simulink library "NREL_Diesel_Genset_lib"  (Simulink 8.1)
settings: Solver=ode45  StartTime=0.0  StopTime=10.0  RelTol=1e-3
values from neighbouring files (symbols this model uses):
  T3dend = [ 1.0000   -0.9913 ]    [initGTS.m]
  T3numd = [ 0    0.0087 ]    [initGTS.m]
  T4numd = [ 27.7778  -27.7237 ]    [initGTS.m]
undefined symbols (not defined in the file or in its folder): DiscIntNeverNeededParam, Efd0, Efd1, Efd2, GP, Ka, Ke, Kf, SeEfd1, SeEfd2, Ta, Te, Tf, Ts, VR0, VRmax, VRmin
libraries: simulink x17, powerlib x9, powerlib_extras x2, powerlib_models x1
(part 2 of 2)

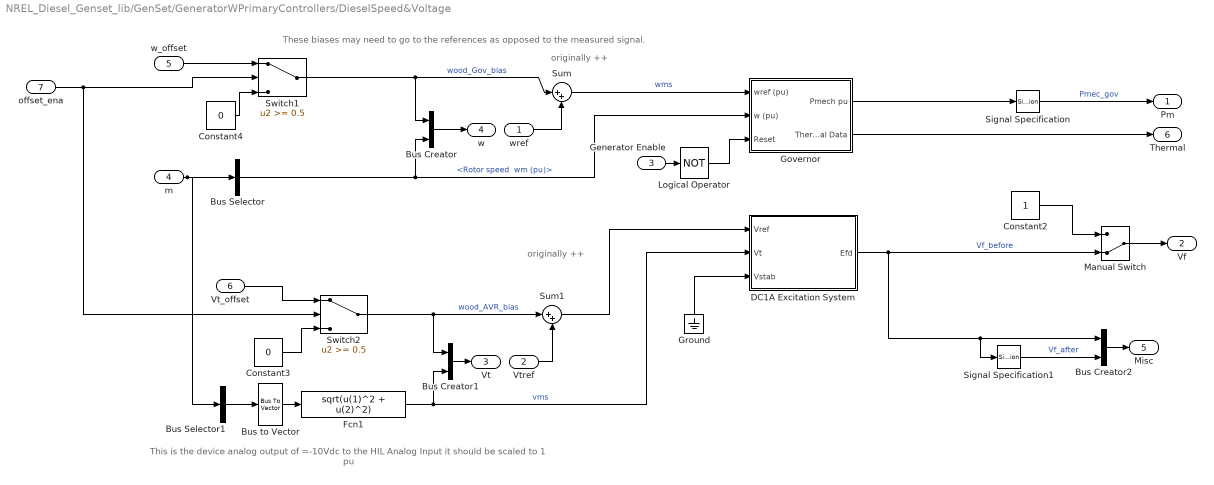
== system NREL_Diesel_Genset_lib/GenSet/GeneratorWPrimaryControllers/DieselSpeed&Voltage ==
  note: originally ++
  note: originally ++
  note: These biases may need to
      | go to the references as opposed
      | to the measured signal.
  note: This is the device analog output of =-10Vdc to
      | the HIL Analog Input it should be scaled to 1 pu
  wref : Inport  SampleTime=Ts
  Vtref : Inport  Port=2  SampleTime=Ts
  Generator Enable : Inport  Port=3  SampleTime=Ts
  m : Inport  Port=4  SampleTime=Ts
  w_offset : Inport  Port=5
  Vt_offset : Inport  Port=6
  offset_ena : Inport  Port=7
  Bus Creator : BusCreator  Inputs=2
  Bus Creator1 : BusCreator  Inputs=2
  Bus Creator2 : BusCreator  Inputs=2
  Bus Selector : BusSelector  OutputSignals="Mechanical.Rotor speed  wm (pu)"
  Bus Selector1 : BusSelector  OutputSignals="dq0 components.Stator voltage  vd (pu),dq0 components.Stator voltage  vq (pu)"  OutputAsBus=on
  Bus to Vector : BusToVector
  Constant2 : Constant
  Constant3 : Constant  Value=0
  Constant4 : Constant  Value=0
  DC1A Excitation System : Subsystem  mask(DC1A Excitation System){Tr=GP.Ex.Tr, KaTa=GP.Ex.Regulator, VRminmax=[0 8], KfTf=GP.Ex.Damping, TbTc=[0 0], KeTe=GP.Ex.Exciter, Efd12=[6.83 6.08], SeEfd12=[ 0.132 0.062], v0=[0 0], TsBlock=Ts}
      mask prompts: Tr "Low-pass filter time constant Tr(s):"; KaTa "Voltage regulator gain and time constant [Ka Ta(s)]:"; VRminmax "Voltage regulator output limits [VRmin(pu) VRmax(pu)]:"; KfTf "Damping filter gain and time constant [Kf Tf(s)]:"; TbTc "Transient gain reduction lead and lag time constants [Tb(s) Tc(s)]:"; KeTe "Exciter gain and time constant [Ke Te(s)]:"; Efd12 "Field voltage values [Efd1(pu) Efd2(pu)]:"; SeEfd12 "Exciter saturation function values [SeEfd1(pu) SeEfd2(pu)]:"; v0 "Initial values of terminal voltage and field voltage [Vt0(pu) Efd0(pu)]:"; TsBlock "Sample time:"
      mask help: Implements a synchronous machine voltage regulator and exciter based on the IEEE type DC1A excitation system model. The output is the field voltage to apply to the Vf input of a Synchronous Machine block. Inputs and output are in p.u.
      mask init:
      | block = gcb;
      | [Ts,BlockChoice,MaskType,Ka,Ta,Ke,Te,Kf,Tf,Tb,Tc,Efd1,Efd2,SeEfd1,SeEfd2,VRmin,VRmax,Vt0,Efd0,VR0] = powericon('ExcitationSystemInit',block,TsBlock,KaTa,KeTe,KfTf,TbTc,Efd12,SeEfd12,VRminmax,v0);
      | %powericon('SetInternalModels','set',block,BlockChoice);
      mask Help: helpview(psbhelp);
      mask Display: color('blue');disp('DC1A')
  Fcn1 : Fcn  Expr=sqrt(u(1)^2 + u(2)^2)
  Governor : Subsystem  BlockChoice=DieselGovernor
      settings: AttributesFormatString=%<BlockChoice>  TemplateBlock=NREL_Diesel_Genset_lib/GovernorConfig  MemberBlocks=DieselGovernor,GEJenbacherJ620
  Ground : Ground
  Logical Operator : Logic  Operator=NOT  AllPortsSameDT=off  OutDataTypeStr=boolean
  Manual Switch : ManualSwitch  CurrentSetting=0
  Signal Specification : SignalSpecification  Dimensions=1
  Signal Specification1 : SignalSpecification  Dimensions=1
  Sum : Sum  Inputs=|++
  Sum1 : Sum  Inputs=|++
  Switch1 : Switch  Threshold=0.5
  Switch2 : Switch  Threshold=0.5
  Pm : Outport
  Vf : Outport  Port=2
  Vt : Outport  Port=3
  w : Outport  Port=4
  Misc : Outport  Port=5
  Thermal : Outport  Port=6
  wires:
  Governor/2(Thermal Data) -> Thermal/1
  Governor/1(Pmech pu) -> Signal Specification/1
  Logical Operator/1 -> Governor/3(Reset)
  Signal Specification1/1 -> Bus Creator2/2  "Vf_after"
  Signal Specification/1 -> Pm/1  "Pmec_gov"
  Sum/1 -> Governor/1(wref (pu))  "wms"
  wref/1 -> Sum/2
  Sum1/1 -> DC1A Excitation System/1(Vref)
  Vtref/1 -> Sum1/2
  Switch2/1 -> Bus Creator1/1, Sum1/1  "wood_AVR_bias"
  Switch1/1 -> Bus Creator/1, Sum/1  "wood_Gov_bias"
  Bus Creator2/1 -> Misc/1
  DC1A Excitation System/1(Efd) -> Manual Switch/2, Bus Creator2/1, Signal Specification1/1  "Vf_before"
  Bus Creator1/1 -> Vt/1
  Bus Creator/1 -> w/1
  Ground/1 -> DC1A Excitation System/3(Vstab)
  Fcn1/1 -> Bus Creator1/2, DC1A Excitation System/2(Vt)  "vms"
  Bus Selector/1 -> Governor/2(w (pu)), Bus Creator/2  "<Rotor speed  wm (pu)>"
  m/1 -> Bus Selector/1, Bus Selector1/1
  Bus Selector1/1 -> Bus to Vector/1
  Bus to Vector/1 -> Fcn1/1
  Generator Enable/1 -> Logical Operator/1
  Constant2/1 -> Manual Switch/1
  Manual Switch/1 -> Vf/1
  Vt_offset/1 -> Switch2/1
  offset_ena/1 -> Switch1/2, Switch2/2
  w_offset/1 -> Switch1/1
  Constant4/1 -> Switch1/3
  Constant3/1 -> Switch2/3

== system NREL_Diesel_Genset_lib/Simulated Generator Controller/Droop/Droop ==
  dfvpq : Inport
  droop : Inport  Port=2
  Demux : Demux
  Demux1 : Demux
  Low Pass{1..4} (4 alike) : DiscreteStateSpace  A=GP.filt.A  B=GP.filt.B  C=GP.filt.C  D=GP.filt.D  SampleTime=-1
  Mux1 : Mux
  Product{,1..3} (4 alike) : Product
  Selector : Selector  InputPortWidth=4  IndexOptions=Index vector (dialog)  Indices=[3 4 1 2]  OutputSizes=1
  dFvpq_out : Outport
  wires:
  Demux/3 -> Low Pass3/1  "p"
  Low Pass2/1 -> Product1/1
  Demux/2 -> Low Pass1/1  "v"
  Demux/1 -> Low Pass2/1  "f"
  Low Pass3/1 -> Product/1
  dfvpq/1 -> Demux/1
  Selector/1 -> dFvpq_out/1
  Low Pass1/1 -> Product3/1
  Demux/4 -> Low Pass4/1  "q"
  Low Pass4/1 -> Product2/1
  Product1/1 -> Mux1/1  "p"
  Product3/1 -> Mux1/2  "q"
  Product/1 -> Mux1/3  "F"
  Product2/1 -> Mux1/4  "v"
  Mux1/1 -> Selector/1
  Demux1/1 -> Product1/2
  Demux1/4 -> Product2/2
  Demux1/3 -> Product/2
  Demux1/2 -> Product3/2
  droop/1 -> Demux1/1

== system NREL_Diesel_Genset_lib/Simulated Generator Controller/Droop/ExtractCoefs ==
  In1 : Inport
  Bus Selector8 : BusSelector  OutputSignals=FP_droop,VQ_droop,FP_droop,VQ_droop
  Mux : Mux
  Out1 : Outport
  wires:
  Bus Selector8/1 -> Mux/1  "<FP_droop>"
  Bus Selector8/4 -> Mux/4  "<VQ_droop>"
  Bus Selector8/2 -> Mux/2  "<VQ_droop>"
  Bus Selector8/3 -> Mux/3  "<FP_droop>"
  Mux/1 -> Out1/1
  In1/1 -> Bus Selector8/1

== system NREL_Diesel_Genset_lib/Simulated Generator Controller/Protection/bitwise_status ==
  note: Constant array has LSB on most left.
  S : Inport
  Bitwise Operator : simulink/Logic and Bit Operations/Bitwise Operator  logicop=OR  UseBitMask=off  NumInputPorts=3  BitMask=bin2dec('11011001')  BitMaskRealWorld=Stored Integer
  Data Type Conversion : DataTypeConversion  OutDataTypeStr=uint16
  Data Type Conversion1 : DataTypeConversion  OutDataTypeStr=double
  Demux : Demux  Outputs=3
  Shift Arithmetic : ArithShift  BitShiftNumber=1  BitShiftDirection=Left
  Shift Arithmetic1 : ArithShift  BitShiftNumber=2  BitShiftDirection=Left
  s : Outport
  wires:
  Data Type Conversion/1 -> Demux/1
  S/1 -> Data Type Conversion/1
  Bitwise Operator/1 -> Data Type Conversion1/1
  Data Type Conversion1/1 -> s/1
  Demux/1 -> Bitwise Operator/1
  Demux/2 -> Shift Arithmetic/1
  Demux/3 -> Shift Arithmetic1/1
  Shift Arithmetic/1 -> Bitwise Operator/2
  Shift Arithmetic1/1 -> Bitwise Operator/3

== system NREL_Diesel_Genset_lib/Simulated Generator Controller/Subsystem/PQ control ==
  P_ref (pu) : Inport
  P (pu) : Inport  Port=2
  Q_ref (pu) : Inport  Port=3
  Q (pu) : Inport  Port=4
  Rst : Inport  Port=5
  w_Rst : Inport  Port=6
  V_Rst : Inport  Port=7
  Discrete PID Controller : simulink/Continuous/PID Controller  Controller=PID  TimeDomain=Discrete-time  SampleTime=-1  IntegratorMethod=Forward Euler  FilterMethod=Forward Euler  Form=Parallel  P=GP.FCtrl.P  I=GP.FCtrl.I  D=0  N=10  InitialConditionSource=external  InitialConditionForIntegrator=0  InitialConditionForFilter=0  ExternalReset=level  LimitOutput=on  UpperSaturationLimit=0.15  LowerSaturationLimit=-0.15  LinearizeAsGain=off  AntiWindupMode=back-calculation  Kb=1  TrackingMode=off  Kt=1  PParamMin=[]  PParamMax=[]  IParamMin=[]  IParamMax=[]  DParamMin=[]  DParamMax=[]  NParamMin=[]  NParamMax=[]  KbParamMin=[]  KbParamMax=[]  KtParamMin=[]  KtParamMax=[]  POutMin=[]  POutMax=[]  IOutMin=[]  IOutMax=[]  DOutMin=[]  DOutMax=[]  NOutMin=[]  NOutMax=[]  KbOutMin=[]  KbOutMax=[]  KtOutMin=[]  KtOutMax=[]  IntegratorOutMin=[]  IntegratorOutMax=[]  FilterOutMin=[]  FilterOutMax=[]  SumOutMin=[]  SumOutMax=[]  SumI1OutMin=[]  SumI1OutMax=[]  SumI2OutMin=[]  SumI2OutMax=[]  SumI3OutMin=[]  SumI3OutMax=[]  SumDOutMin=[]  SumDOutMax=[]  SaturationOutMin=[]  SaturationOutMax=[]  IntegratorContinuousStateAttributes=''  IntegratorStateMustResolveToSignalObject=off  IntegratorRTWStateStorageClass=Auto  FilterContinuousStateAttributes=''  FilterStateMustResolveToSignalObject=off  FilterRTWStateStorageClass=Auto
  Discrete PID Controller1 : simulink/Continuous/PID Controller  Controller=PID  TimeDomain=Discrete-time  SampleTime=-1  IntegratorMethod=Forward Euler  FilterMethod=Forward Euler  Form=Parallel  P=GP.VCtrl.P  I=GP.VCtrl.I  D=0  N=10  InitialConditionSource=external  InitialConditionForIntegrator=0  InitialConditionForFilter=0  ExternalReset=level  LimitOutput=on  UpperSaturationLimit=0.15  LowerSaturationLimit=-0.15  LinearizeAsGain=off  AntiWindupMode=back-calculation  Kb=1  TrackingMode=off  Kt=1  PParamMin=[]  PParamMax=[]  IParamMin=[]  IParamMax=[]  DParamMin=[]  DParamMax=[]  NParamMin=[]  NParamMax=[]  KbParamMin=[]  KbParamMax=[]  KtParamMin=[]  KtParamMax=[]  POutMin=[]  POutMax=[]  IOutMin=[]  IOutMax=[]  DOutMin=[]  DOutMax=[]  NOutMin=[]  NOutMax=[]  KbOutMin=[]  KbOutMax=[]  KtOutMin=[]  KtOutMax=[]  IntegratorOutMin=[]  IntegratorOutMax=[]  FilterOutMin=[]  FilterOutMax=[]  SumOutMin=[]  SumOutMax=[]  SumI1OutMin=[]  SumI1OutMax=[]  SumI2OutMin=[]  SumI2OutMax=[]  SumI3OutMin=[]  SumI3OutMax=[]  SumDOutMin=[]  SumDOutMax=[]  SaturationOutMin=[]  SaturationOutMax=[]  IntegratorContinuousStateAttributes=''  IntegratorStateMustResolveToSignalObject=off  IntegratorRTWStateStorageClass=Auto  FilterContinuousStateAttributes=''  FilterStateMustResolveToSignalObject=off  FilterRTWStateStorageClass=Auto
  Sum : Sum  Inputs=|-+
  Sum1 : Sum  Inputs=|-+
  w_ref (pu) : Outport
  V_ref (pu) : Outport  Port=2
  wires:
  Rst/1 -> Discrete PID Controller1/2, Discrete PID Controller/2
  w_Rst/1 -> Discrete PID Controller/4, Discrete PID Controller/3
  V_Rst/1 -> Discrete PID Controller1/4, Discrete PID Controller1/3
  Sum/1 -> Discrete PID Controller/1
  P (pu)/1 -> Sum/1
  Discrete PID Controller/1 -> w_ref (pu)/1
  P_ref (pu)/1 -> Sum/2
  Sum1/1 -> Discrete PID Controller1/1  "dq"
  Q (pu)/1 -> Sum1/1  "pu"
  Discrete PID Controller1/1 -> V_ref (pu)/1  "v"
  Q_ref (pu)/1 -> Sum1/2  "ref"

== system NREL_Diesel_Genset_lib/GenSet/GeneratorWPrimaryControllers/DieselSpeed&Voltage/DC1A Excitation System ==
  Vref : Inport
  Vt : Inport  Port=2
  Vstab : Inport  Port=3
  Discrete : Subsystem  mask(Excitation System){}
  Efd : Outport
  wires:
  Vref/1 -> Discrete/1(Vref)
  Vt/1 -> Discrete/2(Vt)
  Discrete/1(Efd) -> Efd/1
  Vstab/1 -> Discrete/3(Vstab)

== system NREL_Diesel_Genset_lib/GenSet/GeneratorWPrimaryControllers/DieselSpeed&Voltage/Governor ==
  wref (pu) : Inport
  w (pu) : Inport  Port=2
  Reset : Inport  Port=3
  DieselGovernor : Subsystem  AncestorBlock=NREL_Diesel_Genset_lib/DieselGovernor  mask(Diesel Engine & Governor){K=GP.Gov.Kp, Ta=[0.025 0.0009 0.00574], Tlim=[0 2], Td=0.024, Pm0=0.00005}
      mask prompts: K "Regulator gain K:"; Ta "Actuator time constants [T4 T5 T6] (s) :"; Tlim "Torque limits [Tmin Tmax] (pu) :"; Td "Engine time delay Td (s) :"; Pm0 "Initial value of mechanical power  Pm0 (pu) :"
      mask help:
      | This block implements a diesel engine and governor system:
      | 1st and 2nd inputs: Desired and actual speed (pu)
      | Output: Diesel engine mechanical power.Motor inertia should be combined with generator.
      |
      | Actuator transfer function :
      |      Ha= (1+T4.s) / [ (s (1+T5.s)(1+T6.s) ]
      | Motor :
      |      Time delay Td
      |
      | (See reference in Tutorial Session 5)
  gnd2 : Ground
  Pmech pu : Outport
  Thermal Data : Outport  Port=2
  wires:
  wref (pu)/1 -> DieselGovernor/1(wref (pu))
  w (pu)/1 -> DieselGovernor/2(w (pu))
  Reset/1 -> DieselGovernor/3(Reset)
  DieselGovernor/1(Pmech pu) -> Pmech pu/1
  gnd2/1 -> Thermal Data/1

== system NREL_Diesel_Genset_lib/GenSet/GeneratorWPrimaryControllers/DieselSpeed&Voltage/DC1A Excitation System/Discrete ==
  note: Efd0*Se
  note: __
      |              /
      |           /
      |         /
      |       /
      | __/
  note: VRmin
  note: VRmax
  note: 0
  note: Initial values are shown in blue
  note: Main Regulator
      | Ka/(Ta.s+1)
  note: Efd0
  note: Ke*Efd0
  note: Vt0
  note: Vt0
  note: Efd0
  note: VR0=Efd0*Se+Ke*Efd0
  note: VR0/Ka
  note: VR0/Ka
  note: VR0/Ka
  note: Vt0
  Vref : Inport
  Vt : Inport  Port=2
  Vstab : Inport  Port=3
  1/Te : Gain  Gain=1/Te
  Damping Filter Kf.s/(Tf.s+1) : Subsystem  mask{Kf=Kf, Tf=Tf, X0=Efd0*Kf/Tf}
      mask prompts: Kf "Damping filter gain Kf:"; Tf "Damping filter time constant Tf(s):"; X0 "Initial conditions:"
      mask Display: disp('Kfs\n---\n1+Tfs')
  Discrete-Time Integrator : DiscreteIntegrator  InitialCondition=Efd0  SampleTime=Ts  LimitOutput=on  ICPrevOutput=DiscIntNeverNeededParam  ICPrevScaledInput=DiscIntNeverNeededParam
  Gain3 : Gain  Gain=Ke  SaturateOnIntegerOverflow=on  OutDataTypeStr=Inherit: Same as input  ParamDataTypeStr=Inherit: Same as input
  Low Pass Filter 1/(Tr.s+1) : powerlib_models/Discrete/Excitation_System/Low Pass Filter 1 // (tr.s +1) (with IC)  FilterType=Lowpass  Tc=Tr  Ts=Ts  Initialize=on  Vac_Init=[0 0 60]  Vdc_Init=Vt0  PlotResponse=off  param1=[1 500 0.1]
  Saturation Vx=Efd*Se[Efd] : Subsystem  mask{Efd12=[Efd1 Efd2], SeEfd12=[SeEfd1 SeEfd2]}
      mask prompts: Efd12 "Field voltage values [Efd1(pu) Efd2(pu)]:"; SeEfd12 "Exciter saturation function values [SeEfd1(pu) SeEfd2(pu)]:"
      mask init:
      | Efd1 = Efd12(1);Efd2 = Efd12(2);
      | SeEfd1 = SeEfd12(1);SeEfd2 = SeEfd12(2);
  Sum : Sum  Inputs=++-+-  SaturateOnIntegerOverflow=on  InputSameDT=on  OutDataTypeStr=Inherit: Same as first input
  Sum1 : Sum  Inputs=|+-
  Sum2 : Sum  Inputs=|++
  Transient Gain Reduction (Tc.s+1)/(Tb.s+1) : powerlib_extras/Discrete  Control Blocks/Discrete Lead-Lag  T1=Tc  T2=Tb  V_Init=VR0/Ka  Ts=Ts
  VR0/Ka : Constant  Value=VR0/Ka
  Vaminmax : Subsystem  mask{Ka=Ka, Ta=Ta, VRminmax=[VRmin VRmax], X0=VR0}
      mask prompts: Ka "Voltage regulator gain Ka:"; Ta "Voltage regulator time constant Ta(s):"; VRminmax "Voltage regulator output limits [VRmin(pu) VRmax(pu)]:"; X0 "Initial conditions:"
      mask init:
      | VRmin=VRminmax(1);VRmax=VRminmax(2);
      mask Display: disp('Ka\n---\n1+Tas')
  Efd : Outport
  wires:
  Damping Filter Kf.s/(Tf.s+1)/1(y) -> Sum/5  "Vf"
  Saturation Vx=Efd*Se[Efd]/1(Vx) -> Sum2/1  "Vx"
  Vaminmax/1(y) -> Sum1/1  "VR"
  Sum/1 -> Transient Gain Reduction (Tc.s+1)/(Tb.s+1)/1
  Transient Gain Reduction (Tc.s+1)/(Tb.s+1)/1 -> Vaminmax/1(u)
  Sum2/1 -> Sum1/2  "Vfe"
  Sum1/1 -> 1/Te/1  "Vf"
  Discrete-Time Integrator/1 -> Gain3/1, Damping Filter Kf.s/(Tf.s+1)/1(u), Saturation Vx=Efd*Se[Efd]/1(Efd), Efd/1  "Efd"
  1/Te/1 -> Discrete-Time Integrator/1
  Vref/1 -> Sum/1
  VR0/Ka/1 -> Sum/2
  Low Pass Filter 1/(Tr.s+1)/1 -> Sum/3  "Vt"
  Vstab/1 -> Sum/4
  Gain3/1 -> Sum2/2
  Vt/1 -> Low Pass Filter 1/(Tr.s+1)/1  "Vt"

== system NREL_Diesel_Genset_lib/GenSet/GeneratorWPrimaryControllers/DieselSpeed&Voltage/Governor/DieselGovernor ==
  note: ACTUATOR
  wref (pu) : Inport
  w (pu) : Inport  Port=2
  Reset : Inport  Port=3
  Damping due to pumping losses : Gain  Gain=0.3
  Discrete PID Controller : simulink/Continuous/PID Controller  Controller=PD  TimeDomain=Discrete-time  SampleTime=-1  IntegratorMethod=Forward Euler  FilterMethod=Forward Euler  Form=Parallel  P=1  I=0  D=0.5  N=10000  InitialConditionSource=internal  InitialConditionForIntegrator=0  InitialConditionForFilter=0  ExternalReset=level  ZeroCross=off  LimitOutput=off  UpperSaturationLimit=.5  LowerSaturationLimit=-.5  LinearizeAsGain=off  AntiWindupMode=none  Kb=1  TrackingMode=off  Kt=1  PParamMin=[]  PParamMax=[]  IParamMin=[]  IParamMax=[]  DParamMin=[]  DParamMax=[]  NParamMin=[]  NParamMax=[]  KbParamMin=[]  KbParamMax=[]  KtParamMin=[]  KtParamMax=[]  POutMin=[]  POutMax=[]  IOutMin=[]  IOutMax=[]  DOutMin=[]  DOutMax=[]  NOutMin=[]  NOutMax=[]  KbOutMin=[]  KbOutMax=[]  KtOutMin=[]  KtOutMax=[]  IntegratorOutMin=[]  IntegratorOutMax=[]  FilterOutMin=[]  FilterOutMax=[]  SumOutMin=[]  SumOutMax=[]  SumI1OutMin=[]  SumI1OutMax=[]  SumI2OutMin=[]  SumI2OutMax=[]  SumI3OutMin=[]  SumI3OutMax=[]  SumDOutMin=[]  SumDOutMax=[]  SaturationOutMin=[]  SaturationOutMax=[]  IntegratorContinuousStateAttributes=''  IntegratorStateMustResolveToSignalObject=off  IntegratorRTWStateStorageClass=Auto  FilterContinuousStateAttributes=''  FilterStateMustResolveToSignalObject=off  FilterRTWStateStorageClass=Auto
  Discrete-Time Integrator : DiscreteIntegrator  IntegratorMethod=Integration: Backward Euler  ExternalReset=level  InitialCondition=Pm0  SampleTime=-1  LimitOutput=on  UpperSaturationLimit=Tlim(2)  LowerSaturationLimit=Tlim(1)  ICPrevOutput=DiscIntNeverNeededParam  ICPrevScaledInput=DiscIntNeverNeededParam
  ENGINE Td : TransportDelay  DelayTime=Td  InitialOutput=Pm0  BufferSize=7168
  Gain K : Gain  Gain=K  SaturateOnIntegerOverflow=on  OutDataTypeStr=Inherit: Same as input  ParamDataTypeStr=Inherit: Same as input
  Product : Product  SaturateOnIntegerOverflow=on  InputSameDT=on  OutDataTypeStr=Inherit: Same as first input
  Product1 : Product
  Sum : Sum  Inputs=+-  SaturateOnIntegerOverflow=on  InputSameDT=on  OutDataTypeStr=Inherit: Same as first input
  Sum1 : Sum  Inputs=|+-
  TF3 : DiscreteTransferFcn  Numerator=T3numd  Denominator=T3dend  SampleTime=Ts  RndMeth=Nearest
  TF4 : DiscreteTransferFcn  Numerator=T4numd  Denominator=T3dend  SampleTime=Ts
  Pmech pu : Outport
  wires:
  Reset/1 -> Discrete PID Controller/2, Discrete-Time Integrator/2
  TF4/1 -> TF3/1
  TF3/1 -> Discrete-Time Integrator/1
  Discrete-Time Integrator/1 -> ENGINE Td/1  "Torque"
  Product/1 -> Sum1/1
  wref (pu)/1 -> Sum/1
  ENGINE Td/1 -> Product/1
  Gain K/1 -> TF4/1
  Sum/1 -> Discrete PID Controller/1
  Discrete PID Controller/1 -> Gain K/1
  w (pu)/1 -> Sum/2, Product1/1, Product1/2, Product/2
  Damping due to pumping losses/1 -> Sum1/2
  Product1/1 -> Damping due to pumping losses/1
  Sum1/1 -> Pmech pu/1

== system NREL_Diesel_Genset_lib/GenSet/GeneratorWPrimaryControllers/DieselSpeed&Voltage/DC1A Excitation System/Discrete/Damping Filter Kf.s/(Tf.s+1) ==
  note: Efd0
  note: Efd0*Kf/Tf
  note: 0
  u : Inport
  Discrete 1st-Order Filter : powerlib_extras/Discrete  Control Blocks/Discrete 1st-Order Filter  FilterType=Highpass  Tc=Tf  Ts=Ts  Initialize=on  Vac_Init=[0 0 60]  Vdc_Init=Efd0*Kf/Tf  PlotResponse=off  param1=[1 500 0.1]
  Gain2 : Gain  Gain=Kf/Tf  SaturateOnIntegerOverflow=on  OutDataTypeStr=Inherit: Same as input  ParamDataTypeStr=Inherit: Same as input
  y : Outport
  wires:
  u/1 -> Gain2/1
  Discrete 1st-Order Filter/1 -> y/1
  Gain2/1 -> Discrete 1st-Order Filter/1

== system NREL_Diesel_Genset_lib/GenSet/GeneratorWPrimaryControllers/DieselSpeed&Voltage/DC1A Excitation System/Discrete/Saturation Vx=Efd*Se[Efd] ==
  Efd : Inport
  Lookup Table : Lookup  InputValues=[0 Efd2 Efd1]  Table=[0 SeEfd2 SeEfd1]
  Product : Product  RndMeth=Zero
  Vx : Outport
  wires:
  Efd/1 -> Product/1, Lookup Table/1
  Product/1 -> Vx/1
  Lookup Table/1 -> Product/2

== system NREL_Diesel_Genset_lib/GenSet/GeneratorWPrimaryControllers/DieselSpeed&Voltage/DC1A Excitation System/Discrete/Vaminmax ==
  note: VR0
  note: 0
  note: VR0
  note: VR0
  note: VR0/Ka
  u : Inport
  Discrete-Time Integrator : DiscreteIntegrator  InitialCondition=VR0  SampleTime=Ts  LimitOutput=on  UpperSaturationLimit=VRmax  LowerSaturationLimit=VRmin  ICPrevOutput=DiscIntNeverNeededParam  ICPrevScaledInput=DiscIntNeverNeededParam
  Gain1 : Gain  Gain=1/Ta  SaturateOnIntegerOverflow=on  OutDataTypeStr=Inherit: Same as input  ParamDataTypeStr=Inherit: Same as input
  Gain2 : Gain  Gain=Ka  SaturateOnIntegerOverflow=on  OutDataTypeStr=Inherit: Same as input  ParamDataTypeStr=Inherit: Same as input
  Sum : Sum  Inputs=|+-  SaturateOnIntegerOverflow=on  InputSameDT=on  OutDataTypeStr=Inherit: Same as first input
  y : Outport
  wires:
  Gain1/1 -> Discrete-Time Integrator/1
  Gain2/1 -> Sum/1
  Discrete-Time Integrator/1 -> Sum/2, y/1
  Sum/1 -> Gain1/1
  u/1 -> Gain2/1
